simulink model "model_freq_response"  (R2016a)
settings: Solver=VariableStepAuto  StartTime=0.0  StopTime=20  MaxStep=1e-2  RelTol=1e-3
libraries: simulink x1
settings Model: Creator=alexalcocer  LastModifiedBy=alexalcocer

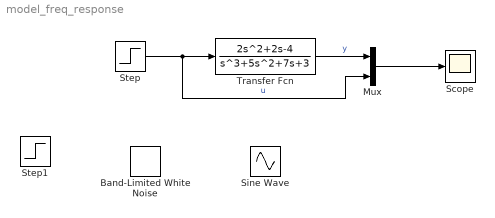
== system model_freq_response ==
  Band-Limited White Noise : simulink/Sources/Band-Limited White Noise  Cov=[0.1]  Ts=0.1  seed=[23341]
  Mux : Mux  Inputs=2
  Scope : Scope
  Sine Wave : Sin  SampleTime=0
  Step : Step  SampleTime=0
  Step1 : Step  SampleTime=0
  Transfer Fcn : TransferFcn  Numerator=[2 2 -4]  Denominator=[1 5 7 3]
  wires:
  Mux/1 -> Scope/1
  Transfer Fcn/1 -> Mux/1  "y"
  Step/1 -> Transfer Fcn/1, Mux/2  "u"
